simulink model "current_control_current_limit_smart_stop"  (R2022b)
settings: Solver=VariableStepAuto  StartTime=0.0  StopTime=10  RelTol=1e-3
libraries: spsCurrentMeasurementLib x4, spsSeriesRLCBranchLib x3, spsVoltageMeasurementLib x2, spsDCMachineLib x1, spsDCVoltageSourceLib x1, spsDiodeLib x1, spsIGBTLib x1, spsThreePhaseSourceLib x1, spsUniversalBridgeLib x1, spspowerguiLib x1
settings Model: Creator=Lenovo  LastModifiedBy=Lenovo

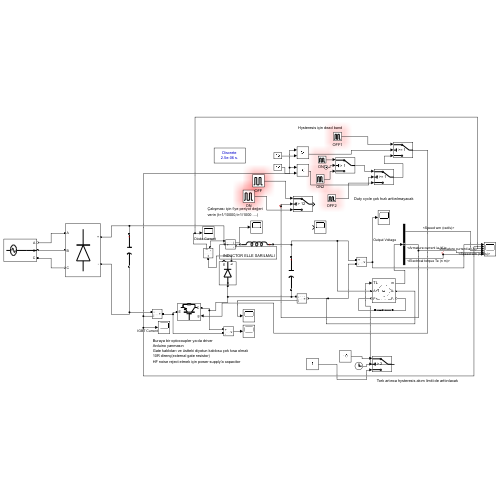
[thumbnail: Simulink's stored preview of the top-level diagram]
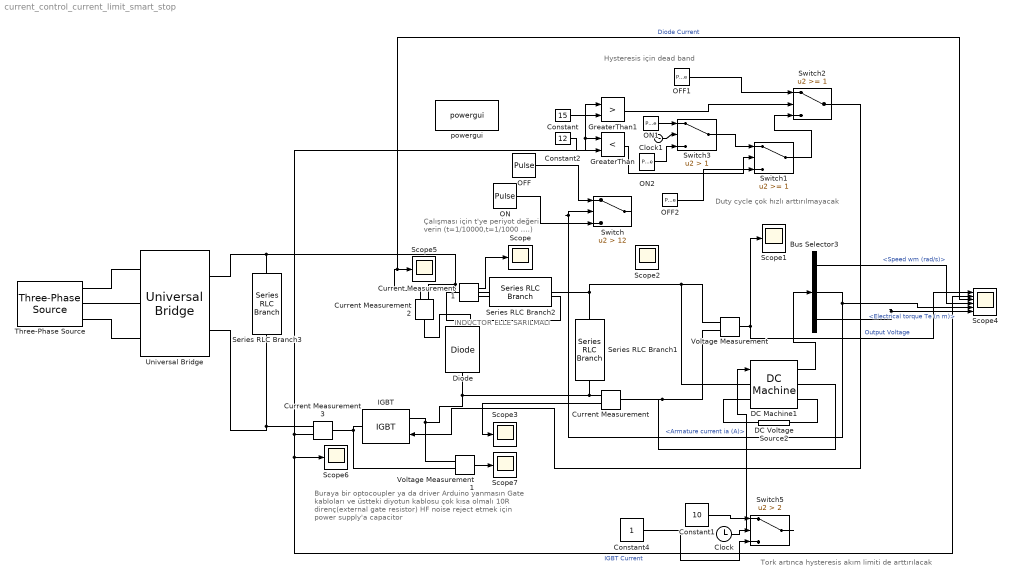
== system current_control_current_limit_smart_stop ==
  note: Çalışması için t'ye periyot değeri
      | verin (t=1/10000,t=1/1000 ....)
  note: INDUCTOR ELLE SARILMALI
  note: Buraya bir optocoupler ya da driver
      | Arduino yanmasın
      | Gate kabloları ve üstteki diyotun kablosu çok kısa olmalı
      | 10R direnç(external gate resistor)
      | HF noise reject etmek için power supply'a capacitor
  note: Tork artınca hysteresis akım limiti de arttırılacak
  note: Duty cycle çok hızlı arttırılmayacak
  note: Hysteresis için dead band
  Bus Selector3 : BusSelector  OutputSignals=Speed wm (rad/s),Armature current ia (A),Electrical torque Te (n m)
  Clock : Clock
  Clock1 : Clock
  Constant : Constant  Value=15
  Constant1 : Constant  Value=10
  Constant2 : Constant  Value=12
  Constant4 : Constant
  Current Measurement{,1..3} (4 alike) : spsCurrentMeasurementLib/Current Measurement  PhasorSimulation=off  OutputType=Complex  PSBequivalent=0
  DC Machine1 : spsDCMachineLib/DC Machine  PresetModel=No  MechanicalLoad=Torque TL  FieldType=Wound  ShowDetailedParameters=on  MeasurementBus=off  RLa="[0.8  0.0125]"  RLf="[210  23]"  Laf=0.9  MachineConstant=Torque constant (N.m/A)  Ke=1.8  Kt=1.8  J=0.4  Bm=0  Tf=0  w0=0  Ifinit=1.42857142857143  TsPowergui=0  TsBlock=-1
  DC Voltage Source2 : spsDCVoltageSourceLib/DC Voltage Source  Amplitude=300  Measurements=None
  Diode : spsDiodeLib/Diode  Ron=0.001  Lon=0  Vf=0.8  IC=0  UseSnubber=0  Rs=0  Cs=0  Measurements=on
  GreaterThan : RelationalOperator  Operator=<  OutDataTypeStr=boolean  RndMeth=Simplest  InputSameDT=off
  GreaterThan1 : RelationalOperator  Operator=>  OutDataTypeStr=boolean  RndMeth=Simplest  InputSameDT=off
  IGBT : spsIGBTLib/IGBT  Ron=0.001  Lon=0  Vf=1  Tf=1e-6  Tt=2e-6  IC=0  Rs=1e5  Cs=inf  Measurements=off
  OFF : DiscretePulseGenerator  PulseType=Time based  Amplitude=0  Period=t
  OFF1 : DiscretePulseGenerator  PulseType=Time based  Amplitude=0  Period=t
  OFF2 : DiscretePulseGenerator  PulseType=Time based  Amplitude=0  Period=t
  ON : DiscretePulseGenerator  PulseType=Time based  Period=t  PulseWidth=10
  ON1 : DiscretePulseGenerator  PulseType=Time based  Period=t  PulseWidth=10
  ON2 : DiscretePulseGenerator  PulseType=Time based  Period=t  PulseWidth=5
  Scope{,1..3,5..7} (7 alike) : Scope
  Scope4 : Scope  NumInputPorts=6
  Series RLC Branch1 : spsSeriesRLCBranchLib/Series RLC Branch  LConnTagsString=__new0  RConnTagsString=__new0  BranchType=C  Resistance=1  Inductance=1e-3  SetiL0=off  InitialCurrent=0  Capacitance=100*1e-6  Setx0=off  InitialVoltage=0  Measurements=None
  Series RLC Branch2 : spsSeriesRLCBranchLib/Series RLC Branch  LConnTagsString=__new0  RConnTagsString=__new0  BranchType=L  Resistance=1  Inductance=1e-3  SetiL0=off  InitialCurrent=0  Capacitance=1e-6  Setx0=off  InitialVoltage=0  Measurements=None
  Series RLC Branch3 : spsSeriesRLCBranchLib/Series RLC Branch  LConnTagsString=__new0  RConnTagsString=__new0  BranchType=C  Resistance=1  Inductance=1e-3  SetiL0=off  InitialCurrent=0  Capacitance=100*1e-6  Setx0=off  InitialVoltage=0  Measurements=None
  Switch : Switch  Criteria=u2 > Threshold  Threshold=12  ZeroCross=off  SaturateOnIntegerOverflow=off  InputSameDT=off
  Switch1 : Switch  Threshold=1  SaturateOnIntegerOverflow=off  InputSameDT=off
  Switch2 : Switch  Threshold=1  SaturateOnIntegerOverflow=off  InputSameDT=off
  Switch3 : Switch  Criteria=u2 > Threshold  Threshold=1  SaturateOnIntegerOverflow=off  InputSameDT=off
  Switch5 : Switch  Criteria=u2 > Threshold  Threshold=2  SaturateOnIntegerOverflow=off  InputSameDT=off
  Three-Phase Source : spsThreePhaseSourceLib/Three-Phase Source  InternalConnection=Y  VoltagePhases=off  Voltage=148.1  PhaseAngle=0  Voltage_phases=[25e3 25e3 25e3]/sqrt(3)  PhaseAngles_phases=[0 -120 +120]  Frequency=50  NonIdealSource=off  SpecifyImpedance=off  Resistance=0.8929  Inductance=16.58e-3  ShortCircuitLevel=100e6  BaseVoltage=25e3  XRratio=7  BusType=swing  Pref=10e3  Qref=0  Prefabc=[10e3, 10e3, 10e3]  Qrefabc=[0, 0, 0]  Qmin=-inf  Qmax=inf
  Universal Bridge : spsUniversalBridgeLib/Universal Bridge  Arms=3  SnubberResistance=1e5  SnubberCapacitance=inf  Device=Diodes  Ron=1e-3  Lon=0  ForwardVoltages="[  0  0  ]"  ForwardVoltage=0  GTOparameters=[ 10e-6 , 20e-6 ]  IGBTparameters=[ 1e-6 , 2e-6 ]  Measurements=None  Measurements_2=None  converterType=Rectifier
  Voltage Measurement : spsVoltageMeasurementLib/Voltage Measurement  PhasorSimulation=off  OutputType=Complex  PSBequivalent=0
  Voltage Measurement1 : spsVoltageMeasurementLib/Voltage Measurement  PhasorSimulation=off  OutputType=Complex  PSBequivalent=0
  powergui : spspowerguiLib/powergui  Priority=1  SimulationMode=Discrete  SampleTime=25*1e-7  frequency=60  Iterations=50  frequencyindice=0  Pbase=100e6  ErrMax=1e-4  UnitsV=kV  UnitsW=MW  buscounter=0  FunctionMessages=off  echomessages=off  EnableUseOfTLC=off  CurrentSourceSwitches=off  DisableSnubberDevices=off  DisableRonSwitches=off  DisableVfSwitches=off  DisplayEquations=off  AutomaticDiscreteSolvers=off  SolverType=Tustin/Backward Euler (TBE)  Interpol=off  ExternalGateDelay=off  methode=off  Ts=100  x0status=blocks  SPID=on  SwTol=0  HookPort=off  NonlinearTolerance=1e-4  nMaxIteration=100  ContinueOnMaxIteration=off  RestoreLinks=warning  ResistiveCurrentMeasurement=off  Frange=[0:2:500]  Ylog=off  Xlog=on  ShowGrid=off  save=off  variable=ZData  structure=0  ZoomFFT=off  StartTime=0.0  cycles=1  DisplayStyle=1  fundamental=60  FreqAxis=off  MaxFrequency=1000  frequencyindicesteady=1  RmsSteady=1  display=off
  wires:
  Current Measurement/1 -> Scope3/1
  DC Machine1/1 -> Bus Selector3/1
  Bus Selector3/1 -> Scope4/4  "<Speed wm (rad/s)>"
  Bus Selector3/2 -> Switch/2, Scope4/5  "<Armature current ia (A)>"
  Bus Selector3/3 -> Scope4/6  "<Electrical torque Te (n m)>"
  Voltage Measurement/1 -> Scope1/1, Scope4/1  "Output Voltage"
  ON/1 -> Switch/3
  OFF/1 -> Switch/1
  Clock/1 -> Switch5/2
  Constant1/1 -> Switch5/1
  Current Measurement1/1 -> Scope/1
  Current Measurement2/1 -> Scope4/3, Scope5/1  "Diode Current"
  Current Measurement3/1 -> Scope4/2, Scope6/1, GreaterThan1/1, GreaterThan/1  "IGBT Current"
  Constant4/1 -> Switch5/3
  Switch5/1 -> DC Machine1/1
  Voltage Measurement1/1 -> Scope7/1
  Constant/1 -> GreaterThan1/2
  OFF1/1 -> Switch2/1
  Switch1/1 -> Switch2/3
  GreaterThan1/1 -> Switch2/2
  GreaterThan/1 -> Switch1/2
  Switch2/1 -> IGBT/1
  Constant2/1 -> GreaterThan/2
  OFF2/1 -> Switch1/3
  Clock1/1 -> Switch3/2
  ON2/1 -> Switch3/3
  ON1/1 -> Switch3/1
  Switch3/1 -> Switch1/1
  connections:
  Current Measurement/RConn1 -- Series RLC Branch1/RConn1 -- Voltage Measurement1/LConn1 -- IGBT/LConn1 -- Diode/LConn1
  DC Machine1/LConn1 -- Series RLC Branch1/LConn1 -- Series RLC Branch2/LConn1 -- Voltage Measurement/LConn1
  DC Voltage Source2/RConn1 -- DC Machine1/LConn2
  DC Voltage Source2/LConn1 -- DC Machine1/RConn2
  Voltage Measurement/LConn2 -- Current Measurement/LConn1 -- DC Machine1/RConn1
  Three-Phase Source/RConn1 -- Universal Bridge/LConn1
  Three-Phase Source/RConn2 -- Universal Bridge/LConn2
  Three-Phase Source/RConn3 -- Universal Bridge/LConn3
  Universal Bridge/RConn2 -- Current Measurement3/RConn1 -- Series RLC Branch3/RConn1
  Current Measurement1/LConn1 -- Current Measurement2/RConn1 -- Series RLC Branch3/LConn1 -- Universal Bridge/RConn1
  Current Measurement1/RConn1 -- Series RLC Branch2/RConn1
  Current Measurement2/LConn1 -- Diode/RConn1
  Current Measurement3/LConn1 -- Voltage Measurement1/LConn2 -- IGBT/RConn1
